simulink model "testPID"  (R2024b)
settings: Solver=FixedStepAuto  StartTime=0.0  StopTime=10.0  FixedStep=0.01  RelTol=1e-3
model workspace (MAT data in the model file):
  M = 1
  g = 9.8
settings Model: Creator=astro  LastModifiedBy=astro

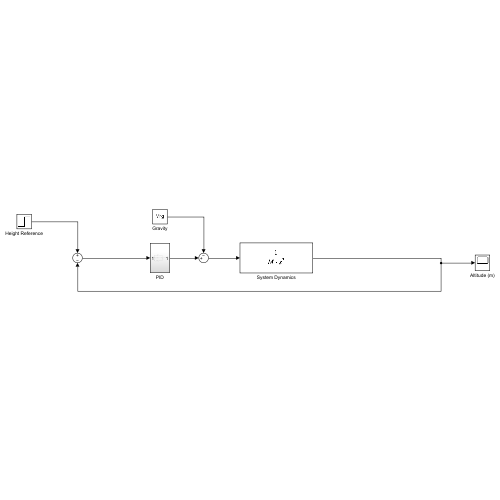
[thumbnail: Simulink's stored preview of the top-level diagram]
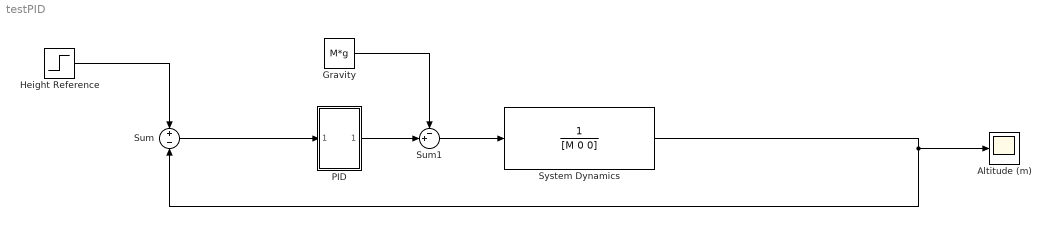
== system testPID ==
  Altitude (m) : Scope
  Gravity : Constant  Value=M*g
  Height Reference : Step  Time=0  SampleTime=0
  PID : Subsystem
  Sum : Sum  Inputs=+|-
  Sum1 : Sum  Inputs=-+|
  System Dynamics : TransferFcn  Denominator=[M 0 0]
  wires:
  Height Reference/1 -> Sum/1
  Sum/1 -> PID/1(In1)
  Sum1/1 -> System Dynamics/1
  System Dynamics/1 -> Sum/2, Altitude (m)/1
  Gravity/1 -> Sum1/1
  PID/1(Out1) -> Sum1/2

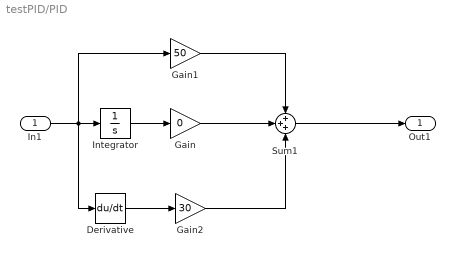
== system testPID/PID ==
  In1 : Inport
  Derivative : Derivative
  Gain : Gain  Gain=0
  Gain1 : Gain  Gain=50
  Gain2 : Gain  Gain=30
  Integrator : Integrator
  Sum1 : Sum  Inputs=+++
  Out1 : Outport
  wires:
  Gain/1 -> Sum1/2
  In1/1 -> Derivative/1, Integrator/1, Gain1/1
  Derivative/1 -> Gain2/1
  Integrator/1 -> Gain/1
  Gain1/1 -> Sum1/1
  Gain2/1 -> Sum1/3
  Sum1/1 -> Out1/1
